simulink model "untitled1"  (R2025b)
settings: Solver=FixedStepAuto  StartTime=0.0  StopTime=30  RelTol=1e-3
libraries: simulink_extras x3
settings Model: Creator=morswin  LastModifiedBy=morswin
settings SolverCC: AutoInsertRateTranBlk=on
settings OptimizationCC: EnhancedBackFolding=on  PassReuseOutputArgsAs=Individual arguments  ZeroExternalMemoryAtStartup=off  ZeroInternalMemoryAtStartup=off  MaxStackSize=64  OptimizeBlockOrder=speed  DifferentSizesBufferReuse=on  OptimizationCustomize=off  EfficientTunableParamExpr=on
settings DebuggingCC: ParameterTunabilityLossMsg=error
settings HardwareCC: ProdBitPerInt=16.0  ProdBitPerPointer=16.0  ProdBitPerSizeT=16.0  ProdBitPerPtrDiffT=16.0  ProdLargestAtomicFloat=None  ProdWordSize=8.0  ProdHWDeviceType=Atmel->AVR
settings SFSimCC: MATLABDynamicMemAlloc=off
settings RTWCC: SystemTargetFile=ert.tlc  TemplateMakefile=ert_default_tmf  Toolchain=Arduino AVR  BuildConfiguration=Faster Runs  Description=Embedded Coder
settings CodeAppCC: ForceParamTrailComments=on  IgnoreCustomStorageClasses=off  OperatorAnnotations=on  SimulinkDataObjDesc=on  SFDataObjDesc=on  InsertBlockDesc=on
settings ERTTargetCC: ExtModeTransport=3.0  ExtModeStaticAlloc=on  ExtModeStaticAllocSize=250.0  ExtModeMexFile=ext_xcp  ExtModeIntrfLevel=Level2 - Open  InlinedParameterPlacement=Hierarchical  ERTCustomFileTemplate=example_file_process.tlc  SupportContinuousTime=on

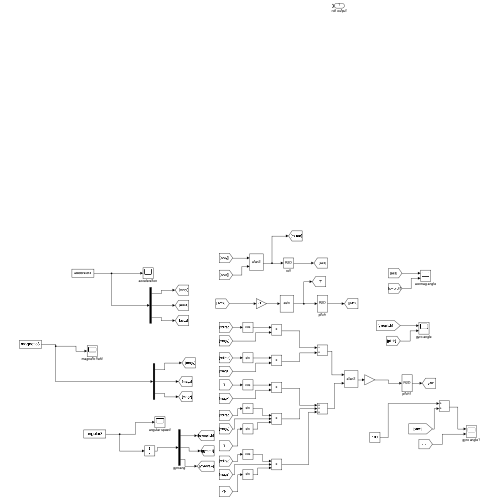
[thumbnail: Simulink's stored preview of the top-level diagram]
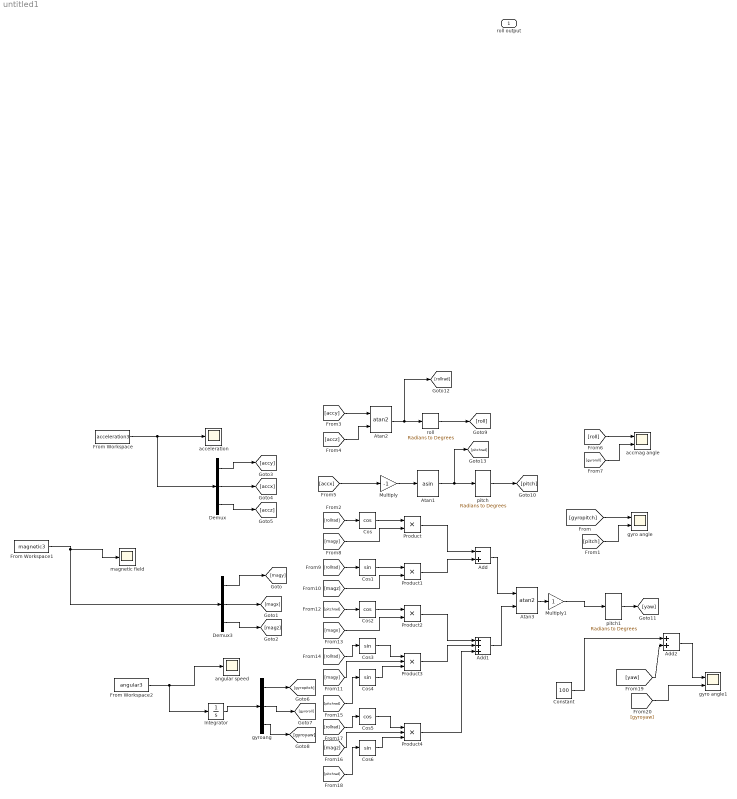
== system untitled1 ==
  Add : Sum  Inputs=-+
  Add1 : Sum  Inputs=+++
  Add2 : Sum
  Atan1 : Trigonometry  Operator=asin
  Atan2 : Trigonometry  Operator=atan2
  Atan3 : Trigonometry  Operator=atan2
  Constant : Constant  Value=100
  Cos : Trigonometry  Operator=cos
  Cos{1,3..4,6} (4 alike) : Trigonometry
  Cos2 : Trigonometry  Operator=cos
  Cos5 : Trigonometry  Operator=cos
  Demux : Demux  Outputs=3
  Demux3 : Demux  Outputs=3
  From Workspace : FromWorkspace  VariableName=acceleration3  SampleTime=0.1
  From Workspace1 : FromWorkspace  VariableName=magnetic3  SampleTime=0.1
  From Workspace2 : FromWorkspace  VariableName=angular3  SampleTime=0.1
  Integrator : Integrator
  Multiply : Gain  Gain=-1
  Multiply1 : Gain
  Product : Product
  Product1 : Product
  Product2 : Product
  Product3 : Product  Inputs=3
  Product4 : Product  Inputs=3
  acceleration : Scope
      settings: ActiveDisplayYMinimum=-1.2818954094057273  ActiveDisplayYMaximum=1.775989632656285
  accmag angle : Scope  NumInputPorts=2
      settings: ActiveDisplayYMinimum=-243.48120331886477  ActiveDisplayYMaximum=221.44822792117074  DataLoggingVariableName=ScopeData4
  angular speed : Scope
      settings: ActiveDisplayYMinimum=-234.74238403439892  ActiveDisplayYMaximum=270.75079730673281  DataLoggingVariableName=ScopeData2
  gyro angle : Scope  NumInputPorts=2
      settings: ActiveDisplayYMinimum=-289.44692166394634  ActiveDisplayYMaximum=339.13692750844524  DataLoggingVariableName=ScopeData3
  gyro angle1 : Scope  NumInputPorts=2
      settings: ActiveDisplayYMinimum=-184.03538179958659  ActiveDisplayYMaximum=571.9226102817147  DataLoggingVariableName=ScopeData5
  gyroang : Demux  Outputs=3
  magnetic field : Scope
      settings: ActiveDisplayYMinimum=0.2503217711232667  ActiveDisplayYMaximum=0.31296781223900094
  pitch : simulink_extras/Transformations/Radians to Degrees
  pitch1 : simulink_extras/Transformations/Radians to Degrees
  roll : simulink_extras/Transformations/Radians to Degrees
  roll output : Outport
  wires:
  Demux3/2 -> [magx]
  [yaw] -> Add2/2
  Product/1 -> Add/1
  Product1/1 -> Add/2
  Atan3/1 -> Multiply1/1
  gyroang/3 -> [gyroyaw]
  [rollrad] -> Cos1/1
  [accx] -> Multiply/1
  [magx] -> Product2/2
  Cos4/1 -> Product3/3
  Demux/2 -> [accx]
  gyroang/2 -> [gyroroll]
  [rollrad] -> Cos3/1
  Product4/1 -> Add1/3
  Demux/3 -> [accz]
  From Workspace1/1 -> Demux3/1, magnetic field/1
  Cos6/1 -> Product4/3
  [gyroyaw] -> gyro angle1/2
  [gyroroll] -> accmag angle/2
  Product2/1 -> Add1/1
  Cos3/1 -> Product3/1
  [accz] -> Atan2/2
  [pitch] -> gyro angle/2
  [rollrad] -> Cos/1
  [roll] -> accmag angle/1
  [magy] -> Product3/2
  From Workspace/1 -> Demux/1, acceleration/1
  [pitchrad] -> Cos2/1
  Add/1 -> Atan3/1
  [accy] -> Atan2/1
  Integrator/1 -> gyroang/1
  [magy] -> Product/2
  [magz] -> Product1/2
  From Workspace2/1 -> Integrator/1, angular speed/1
  Demux/1 -> [accy]
  [rollrad] -> Cos5/1
  Atan1/1 -> [pitchrad], pitch/1
  Multiply1/1 -> pitch1/1
  gyroang/1 -> [gyropitch]
  Atan2/1 -> [rollrad], roll/1
  Cos/1 -> Product/1
  roll/1 -> [roll]
  Multiply/1 -> Atan1/1
  Cos2/1 -> Product2/1
  Product3/1 -> Add1/2
  [pitchrad] -> Cos6/1
  Demux3/3 -> [magz]
  [gyropitch] -> gyro angle/1
  pitch/1 -> [pitch]
  [pitchrad] -> Cos4/1
  Add1/1 -> Atan3/2
  Cos1/1 -> Product1/1
  [magz] -> Product4/2
  Cos5/1 -> Product4/1
  pitch1/1 -> [yaw]
  Demux3/1 -> [magy]
  Add2/1 -> gyro angle1/1
  Constant/1 -> Add2/1
